simulink model "panelSim"  (R2024b)
settings: Solver=ode4  StartTime=0.0  StopTime=0.2  FixedStep=1e-5  RelTol=1e-3  EnableMultiTasking=on
model workspace (MAT data in the model file):
  Temperature = 1
  irradience = 1
undefined symbols (not defined in the file): irradiance, temp
libraries: spsControlledCurrentSourceLib x1, spsDiodeLib x1, spsSeriesRLCBranchLib x1, spsVoltageMeasurementLib x1, sps_lib x1
settings Model: Creator=Prasun  LastModifiedBy=lukel
settings SolverCC: AlgebraicLoopSolver=TrustRegion
settings DataIOCC: LimitDataPoints=on  SaveFormat=Array  ReturnWorkspaceOutputs=off
settings OptimizationCC: LifeSpan=inf
settings DebuggingCC: UnderspecifiedInitializationDetection=Classic  MergeDetectMultiDrivingBlocksExec=none  SolverPrmCheckMsg=warning  UnconnectedInputMsg=warning  UnconnectedOutputMsg=warning  UnconnectedLineMsg=warning  StateNameClashWarn=warning  SFUnexpectedBacktrackingDiag=warning  SFNoUnconditionalDefaultTransitionDiag=warning  SFExecutionAtInitializationDiag=none  ArithmeticOperatorsInVariantConditions=warning
settings HardwareCC: ProdBitPerPointer=32  ProdBitPerSizeT=32  ProdBitPerPtrDiffT=32  ProdLargestAtomicFloat=None  ProdIntDivRoundTo=Undefined  ProdEndianess=Unspecified  ProdWordSize=32  ProdHWDeviceType=32-bit Generic
settings ModelReferenceCC: PropagateSignalLabelsOutOfModel=off
settings SFSimCC: SimUseLocalCustomCode=off  CustomCodeUndefinedFunction=UseInterfaceOnly
settings RTWCC: RTWUseLocalCustomCode=off  GPUComputeCapability=3.5
settings CodeAppCC: StateflowObjectComments=on
settings GRTTargetCC: TargetLangStandard=C89/C90 (ANSI)
settings ConfigComp: CovMetricSettings=dw  CovSaveCumulativeToWorkspaceVar=on  CovSaveSingleToWorkspaceVar=on  CovExternalEMLEnable=off
settings SimscapeCC: SimscapeNormalizeSystem=off

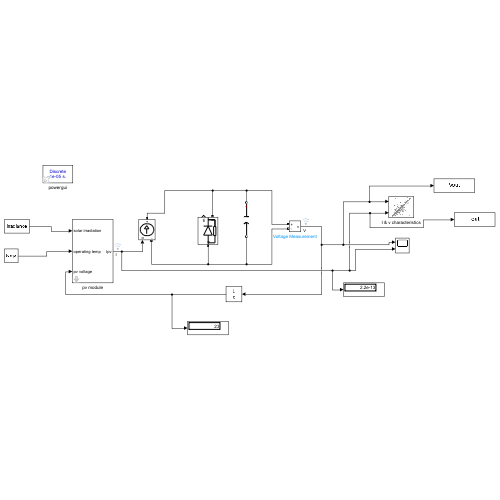
[thumbnail: Simulink's stored preview of the top-level diagram]
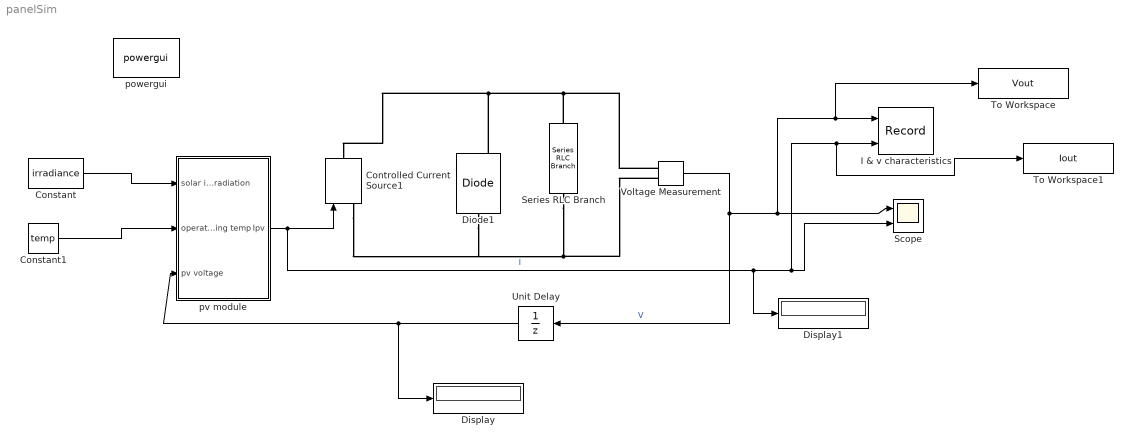
== system panelSim ==
  Constant : Constant  Value=irradiance
  Constant1 : Constant  Value=temp
  Controlled Current Source1 : spsControlledCurrentSourceLib/Controlled Current Source  Initialize=on  Source_Type=AC  Amplitude=0  Phase=0  Frequency=0  Measurements=None
  Diode1 : spsDiodeLib/Diode  Ron=0.001  Lon=0  Vf=0.8  IC=0  UseSnubber=off  Rs=500  Cs=250e-9  Measurements=on
  Display : Display
  Display1 : Display
  I & v characteristics : Record  FileSettingsInternal="{\"entries\":[{\"content\":{\"excelSettings\":{\"content\":{},\"type\":\"Streamout.ExcelSettings\"}},\"type\":\"Streamout.FileSettingStorage\",\"uuid\":\"\"}],\"packageUris\":[\"http:\\/\\/schema.mathworks.com\\/mf0\\/streamout_blocks\\/R2020a\"],\"version\":\"1.0\"}"  Layout=[1 1]  SignalsInternal="{\"entries\":[{\"content\":{\"signals\":[{\"content\":{\"blockPath\":[],\"dimensions\":[1],\"domain\":\"\",\"lineColor\":\"#a2142f\",\"plots\":[ 1 ],\"port\":1,\"sid\":[\"\"],\"signalID\":1,\"signalName\":\"V\"},\"type\":\"RecordBlkView.Signal\",\"uuid\":\"\"},{\"content\":{\"blockPath\":[],\"dimensions\":[1],\"domain\":\"\",\"lineColor\":\"#139fff\",\"plots\":[ 1 ],\"port\":2,\"sid\":[\"\"],\"signalID\":2,\"signalName\":\"I\"},\"type\":\"RecordBlkView.Signal\",\"uuid\":\"\"}]},\"type\":\"RecordBlkView.InputSignals\",\"uuid\":\"\"}],\"packageUris\":[\"http:\\/\\/schema.mathworks.com\\/mf0\\/streamout_blocks\\/R2020a\"],\"version\":\"1.0\"}"  VisualizationBindings="{\"xyplotplugin\":{\"info\":[{\"series\":[{\"bindingParametersList\":[{\"parameter\":\"X-Axis\",\"signalID\":1,\"signalName\":\"V\"},{\"parameter\":\"Y-Axis\",\"signalID\":2,\"signalName\":\"I\"}],\"seriesID\":0}],\"subplotID\":1}]}}"  CompatibilityTag=XY  st=-1
  Scope : Scope  NumInputPorts=2
  Series RLC Branch : spsSeriesRLCBranchLib/Series RLC Branch  LConnTagsString=__new0  RConnTagsString=__new0  BranchType=C  Resistance=1  Inductance=1e-3  SetiL0=off  InitialCurrent=0  Capacitance=1000e-6  Setx0=on  InitialVoltage=0  Measurements=None
  To Workspace : ToWorkspace  VariableName=Vout  SampleTime=-1
  To Workspace1 : ToWorkspace  VariableName=Iout  SampleTime=-1
  Unit Delay : UnitDelay  SampleTime=-1  HasFrameUpgradeWarning=on
  Voltage Measurement : spsVoltageMeasurementLib/Voltage Measurement  PhasorSimulation=off  OutputType=Complex  PSBequivalent=0
  powergui : sps_lib/powergui  Priority=1  SimulationMode=Discrete  SampleTime=1e-5  frequency=60  Iterations=50  frequencyindice=0  Pbase=100e6  ErrMax=1e-4  UnitsV=kV  UnitsW=MW  buscounter=0  FunctionMessages=off  echomessages=off  EnableUseOfTLC=off  CurrentSourceSwitches=off  DisableSnubberDevices=off  DisableRonSwitches=off  DisableVfSwitches=off  DisplayEquations=off  AutomaticDiscreteSolvers=off  SolverType=Tustin  Interpol=off  ExternalGateDelay=off  methode=off  Ts=0  x0status=blocks  SPID=off  SwTol=0  HookPort=off  NonlinearTolerance=1e-4  nMaxIteration=100  ContinueOnMaxIteration=off  RestoreLinks=warning  ResistiveCurrentMeasurement=off  Frange=[0:2:500]  Ylog=off  Xlog=on  ShowGrid=off  save=off  variable=ZData  structure=0  ZoomFFT=off  StartTime=0.0  cycles=1  DisplayStyle=1  fundamental=60  FreqAxis=off  MaxFrequency=1000  frequencyindicesteady=1  RmsSteady=1  display=off
  pv module : Subsystem  mask{Voc=23, Isc=1.2, Ns=36, Np=1, Rsh=1000, Rs=0.0001}
      mask prompts: Voc "open circuit voltage"; Isc "shortcircuit current"; Ns "modules in series"; Np "modules in parallel"; Rsh "shunt resistance"; Rs "series resistance"
  wires:
  Constant/1 -> pv module/1(solar irradiation)
  Constant1/1 -> pv module/2(operating temp)
  Unit Delay/1 -> Display/1, pv module/3(pv voltage)
  pv module/1(Ipv) -> Display1/1, To Workspace1/1, I & v characteristics/2, Scope/2, Controlled Current Source1/1  "I"
  Voltage Measurement/1 -> To Workspace/1, I & v characteristics/1, Scope/1, Unit Delay/1  "V"
  connections:
  Series RLC Branch/RConn1 -- Voltage Measurement/LConn2 -- Diode1/LConn1 -- Controlled Current Source1/LConn1
  Voltage Measurement/LConn1 -- Series RLC Branch/LConn1 -- Diode1/RConn1 -- Controlled Current Source1/RConn1

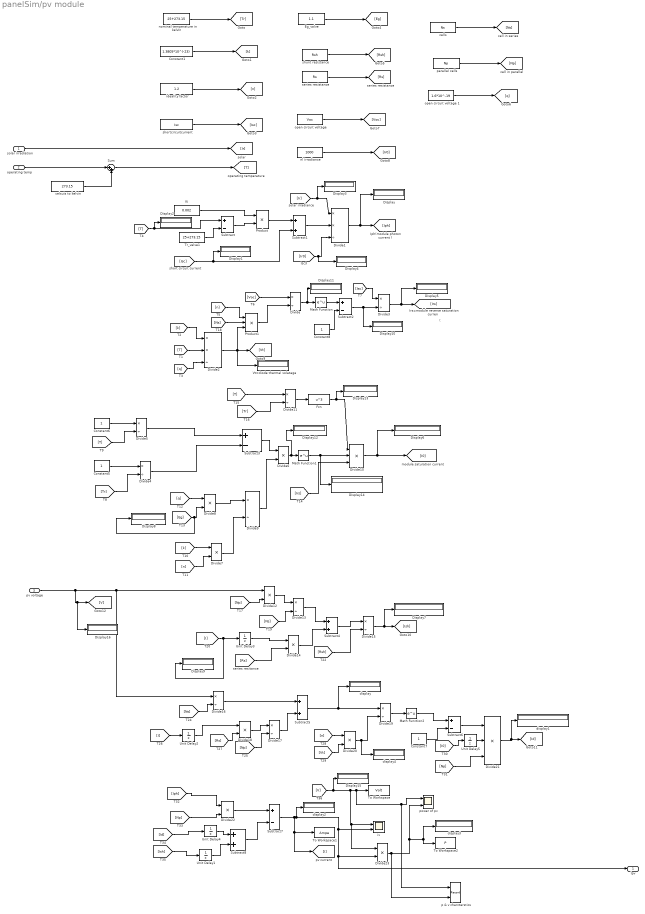
== system panelSim/pv module ==
  note: t
  solar irradiation : Inport
  operating temp : Inport  Port=2
  pv voltage : Inport  Port=3
  Constant1 : Constant  Value=1.3805*10^(-23)
  Constant{5..8} (4 alike) : Constant
  Display{,1..16} (17 alike) : Display
  Divide{,3..5,9,11,13,15..17,19} (11 alike) : Product  Inputs=*/
  Divide1 : Product  Inputs=**/
  Divide10 : Product  Inputs=***
  Divide{6..8,12,14,18,20,22..23} (9 alike) : Product  Inputs=**
  Divide2 : Product  Inputs=**/
  Divide21 : Product  Inputs=***
  "Eg_valve " : Constant  Value=1.1
  Fcn : Fcn  Expr=u^3
  Ki : Constant  Value=0.002
  Math Function : Math  SignedPower=on
  Math Function1 : Math  SignedPower=on
  Math Function2 : Math  SignedPower=on
  Product : Product
  Product1 : Product  Inputs=3
  Subtract{,2..3,6..7} (5 alike) : Sum  Inputs=+-
  Subtract{1,4..5,8} (4 alike) : Sum
  Sum : Sum  Inputs=|++
  To Workspace : ToWorkspace  VariableName=Volt  SaveFormat=Timeseries  SampleTime=-1
  To Workspace1 : ToWorkspace  VariableName=Ampe  SaveFormat=Timeseries  SampleTime=-1
  To Workspace2 : ToWorkspace  VariableName=P  SaveFormat=Timeseries  SampleTime=-1
  Tr_valve1 : Constant  Value=25+273.15
  Unit Delay{1..5} (5 alike) : UnitDelay  SampleTime=-1  HasFrameUpgradeWarning=on
  Vt=diode thermal volatage : Display
  cells : Constant  Value=Ns
  celsuis to kelvin : Constant  Value=273.15
  display{,1..4} (5 alike) : Display
  ideality factor : Constant  Value=1.2
  iv : Scope  NumInputPorts=2
  nl irradiance : Constant  Value=1000
  "nominal temperature in kelvin " : Constant  Value=25+273.15
  "open circuit voltage " : Constant  Value=Voc
  open circuit voltage 1 : Constant  Value=1.6*10^-19
  "p & v charcterstics " : Record  FileSettingsInternal="{\"entries\":[{\"content\":{\"excelSettings\":{\"content\":{},\"type\":\"Streamout.ExcelSettings\"}},\"type\":\"Streamout.FileSettingStorage\",\"uuid\":\"\"}],\"packageUris\":[\"http:\\/\\/schema.mathworks.com\\/mf0\\/streamout_blocks\\/R2020a\"],\"version\":\"1.0\"}"  Layout=[1 1]  SignalsInternal="{\"entries\":[{\"content\":{\"signals\":[{\"content\":{\"blockPath\":[],\"dimensions\":[1],\"domain\":\"\",\"lineColor\":\"#a2142f\",\"plots\":[ 1 ],\"port\":1,\"sid\":[\"\"],\"signalID\":1,\"signalName\":\"T36\"},\"type\":\"RecordBlkView.Signal\",\"uuid\":\"\"},{\"content\":{\"blockPath\":[],\"dimensions\":[1],\"domain\":\"\",\"lineColor\":\"#139fff\",\"plots\":[ 1 ],\"port\":2,\"sid\":[\"\"],\"signalID\":2,\"signalName\":\"Divide23\"},\"type\":\"RecordBlkView.Signal\",\"uuid\":\"\"}]},\"type\":\"RecordBlkView.InputSignals\",\"uuid\":\"\"}],\"packageUris\":[\"http:\\/\\/schema.mathworks.com\\/mf0\\/streamout_blocks\\/R2020a\"],\"version\":\"1.0\"}"  VisualizationBindings="{\"xyplotplugin\":{\"info\":[{\"series\":[{\"bindingParametersList\":[{\"parameter\":\"X-Axis\",\"signalID\":1,\"signalName\":\"T36\"},{\"parameter\":\"Y-Axis\",\"signalID\":2,\"signalName\":\"Divide23\"}],\"seriesID\":0}],\"subplotID\":1}]}}"  CompatibilityTag=XY  st=-1
  parallel cells : Constant  Value=Np
  power of pv : Scope  NumInputPorts=2
  series resistance : Constant  Value=Rs
  "shortcircuitcurrent " : Constant  Value=Isc
  "shunt resistance " : Constant  Value=Rsh
  Ipv : Outport
  wires:
  Subtract7/1 -> display2/1, Ipv/1, Divide23/2, iv/2, To Workspace1/1, [I]
  Divide10/1 -> Display6/1, [I0]
  Math Function/1 -> Subtract2/1
  Divide6/1 -> Display12/1, Math Function1/1
  [n] -> Product1/1
  [n] -> Divide7/2
  Constant8/1 -> Subtract2/2
  Constant5/1 -> Divide4/1
  [T] -> Divide11/1
  Subtract5/1 -> display/1, Divide19/1
  [Np] -> Divide17/2
  Divide11/1 -> Fcn/1
  [V] -> Display15/1, Divide23/1, iv/1, "p & v charcterstics "/1, power of pv/1, To Workspace/1
  Product/1 -> Subtract1/1
  Math Function1/1 -> Display14/1, Divide10/2
  Constant7/1 -> Subtract6/2
  [k] -> Divide2/1
  [Tr] -> Divide11/2
  "Eg_valve "/1 -> [Eg]
  Divide17/1 -> Subtract5/2
  [q] -> Divide2/3
  ideality factor/1 -> [n]
  Divide12/1 -> Divide13/1
  "shortcircuitcurrent "/1 -> [Isc]
  [Eg] -> Display8/1, Divide8/2
  [Isc] -> Divide3/1
  Ki/1 -> Product/1
  Subtract/1 -> Product/2
  [Tr] -> Divide4/2
  [q] -> Divide8/1
  Product1/1 -> Divide/2
  Subtract6/1 -> Divide21/1
  Constant1/1 -> [k]
  [n] -> Divide20/1
  solar irradiation/1 -> [Ir]
  Divide14/1 -> Subtract4/2
  Math Function2/1 -> Subtract6/1
  [Vt] -> Divide20/2
  Divide1/1 -> Display/1, [Iph]
  Subtract8/1 -> Subtract7/2
  Divide16/1 -> Subtract5/1
  [T] -> Divide2/2
  Divide15/1 -> Display7/1, [Ish]
  Divide18/1 -> Divide17/1
  [Rs] -> Divide18/2
  Subtract2/1 -> Display10/1, Divide3/2
  [Rsh] -> Divide15/2
  Fcn/1 -> Display13/1, Divide10/1
  Divide3/1 -> Display5/1, [Irs]
  pv voltage/1 -> Divide16/1, Divide12/1, Display16/1, [V]
  [Ir0] -> Display4/1, Divide1/3
  [Ns] -> Divide13/2
  Divide13/1 -> Subtract4/1
  [Np] -> Divide21/3
  Divide/1 -> Display11/1, Math Function/1
  [T] -> Display2/1, Subtract/1
  [Irs] -> Divide10/3
  [Np] -> Divide22/2
  Divide21/1 -> display1/1, [Id]
  Divide2/1 -> Product1/3, Vt=diode thermal volatage/1, [Vt]
  Divide22/1 -> Subtract7/1
  [Voc] -> Divide/1
  "shunt resistance "/1 -> [Rsh]
  Divide9/1 -> Divide6/2
  Tr_valve1/1 -> Subtract/2
  [k] -> Divide7/1
  Divide20/1 -> display4/1, Divide19/2
  Divide19/1 -> Math Function2/1
  "open circuit voltage "/1 -> [Voc]
  Subtract4/1 -> Divide15/1
  [Np] -> Divide12/2
  [Ns] -> Divide16/2
  [Rs] -> Divide14/2
  Subtract3/1 -> Divide6/1
  [Isc] -> Display1/1, Subtract1/2
  Subtract1/1 -> Divide1/2
  [Ir] -> Display3/1, Divide1/1
  "nominal temperature in kelvin "/1 -> [Tr]
  [Iph] -> Divide22/1
  [Ish] -> Unit Delay1/1
  Unit Delay1/1 -> Subtract8/2
  [I] -> Unit Delay2/1
  Unit Delay2/1 -> Divide18/1
  open circuit voltage 1/1 -> [q]
  cells/1 -> [Ns]
  parallel cells/1 -> [Np]
  series resistance/1 -> [Rs]
  nl irradiance/1 -> [Ir0]
  [I] -> Display9/1, Unit Delay3/1
  [Ns] -> Product1/2
  Constant6/1 -> Divide5/1
  [T] -> Divide5/2
  Divide8/1 -> Divide9/1
  Divide7/1 -> Divide9/2
  Divide5/1 -> Subtract3/1
  Divide4/1 -> Subtract3/2
  Unit Delay3/1 -> Divide14/1
  [Id] -> Unit Delay4/1
  Unit Delay4/1 -> Subtract8/1
  Unit Delay5/1 -> Divide21/2
  [I0] -> Unit Delay5/1
  operating temp/1 -> Sum/1
  Sum/1 -> [T]
  celsuis to kelvin/1 -> Sum/2
  Divide23/1 -> "p & v charcterstics "/2, display3/1, To Workspace2/1, power of pv/2
